simulink model "regulacja_pid"  (R2016b)
settings: Solver=VariableStepAuto  StartTime=0.0  StopTime=Tsym  RelTol=1e-3
undefined symbols (not defined in the file): D_12, D_21, decouplingEnabled, deltaFd, deltah, deltaT, deltaTc, deltaTd, deltaTh, disturbanceTime, enable_cross_tf, Fc_max, Fc_min, Fh_max, Fh_min, G1, h0, h_step_down_time, h_step_up_time, Kd, pid_ovation_h, pid_ovation_T, T0, T_step_down_time, T_step_up_time, Tp_pid
settings Model: Creator=Luke  LastModifiedBy=Luke

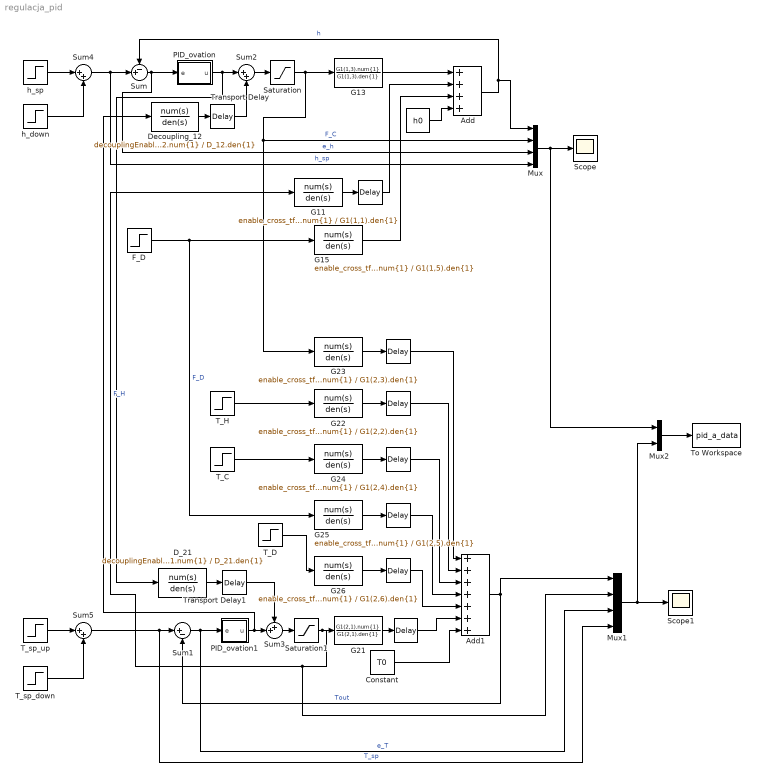
== system regulacja_pid ==
  " " : Constant  Value=h0
  "  " : TransportDelay  DelayTime=G1(2,1).ioDelay
  "   " : TransportDelay  DelayTime=G1(2,3).ioDelay
  "    " : TransportDelay  DelayTime=G1(2,2).ioDelay
  "     " : TransportDelay  DelayTime=G1(2,4).ioDelay
  "       " : TransportDelay  DelayTime=G1(2,5).ioDelay
  "        " : TransportDelay  DelayTime=G1(2,6).ioDelay
  "           " : TransportDelay  DelayTime=G1(1,1).IOdelay
  Add : Sum  Inputs=++++
  Add1 : Sum  Inputs=+++++++
  Constant : Constant  Value=T0
  D_21 : TransferFcn  Numerator=decouplingEnabled * D_21.num{1}  Denominator=D_21.den{1}
  Decoupling_12 : TransferFcn  Numerator=decouplingEnabled * D_12.num{1}  Denominator=D_12.den{1}
  F_D : Step  Time=1000  After=deltaFd  SampleTime=disturbanceTime
  G11 : TransferFcn  Numerator=enable_cross_tf * G1(1,1).num{1}  Denominator=G1(1,1).den{1}
  G13 : TransferFcn  Numerator=G1(1,3).num{1}  Denominator=G1(1,3).den{1}
  G15 : TransferFcn  Numerator=enable_cross_tf * G1(1,5).num{1}  Denominator=G1(1,5).den{1}
  G21 : TransferFcn  Numerator=G1(2,1).num{1}  Denominator=G1(2,1).den{1}
  G22 : TransferFcn  Numerator=enable_cross_tf * G1(2,2).num{1}  Denominator=G1(2,2).den{1}
  G23 : TransferFcn  Numerator=enable_cross_tf * G1(2,3).num{1}  Denominator=G1(2,3).den{1}
  G24 : TransferFcn  Numerator=enable_cross_tf * G1(2,4).num{1}  Denominator=G1(2,4).den{1}
  G25 : TransferFcn  Numerator=enable_cross_tf * G1(2,5).num{1}  Denominator=G1(2,5).den{1}
  G26 : TransferFcn  Numerator=enable_cross_tf * G1(2,6).num{1}  Denominator=G1(2,6).den{1}
  Mux : Mux
  Mux1 : Mux
  Mux2 : Mux  Inputs=2
  PID_ovation : Subsystem
  PID_ovation1 : Subsystem
  Saturation : Saturate  UpperLimit=Fc_max  LowerLimit=Fc_min
  Saturation1 : Saturate  UpperLimit=Fh_max  LowerLimit=Fh_min
  Scope : Scope
  Scope1 : Scope
  Sum : Sum  Inputs=-+|
  Sum1 : Sum  Inputs=|+-
  Sum2 : Sum  Inputs=|++
  Sum3 : Sum  Inputs=++|
  Sum4 : Sum  Inputs=|++
  Sum5 : Sum  Inputs=|++
  T_C : Step  After=deltaTc  SampleTime=0
  T_D : Step  After=deltaTd  SampleTime=0
  T_H : Step  After=deltaTh  SampleTime=0
  T_sp_down : Step  Time=T_step_down_time  After=-deltaT  SampleTime=0
  T_sp_up : Step  Time=T_step_up_time  Before=T0  After=T0+deltaT  SampleTime=0
  To Workspace : ToWorkspace  VariableName=pid_a_data  SaveFormat=Timeseries  SampleTime=-1
  Transport Delay : TransportDelay  DelayTime=D_12.IOdelay
  Transport Delay1 : TransportDelay  DelayTime=D_21.IOdelay
  h_down : Step  Time=h_step_down_time  After=-deltah  SampleTime=0
  h_sp : Step  Time=h_step_up_time  Before=h0  After=h0+deltah  SampleTime=0
  wires:
  " "/1 -> Add/4
  Add/1 -> Sum/1, Mux/1  "h"
  G13/1 -> Add/1
  PID_ovation/1(u) -> D_21/1, Sum2/1
  Sum/1 -> PID_ovation/1(e), Mux/3  "e_h"
  Sum4/1 -> Mux/4, Sum/2  "h_sp"
  Mux/1 -> Mux2/1, Scope/1
  G15/1 -> Add/3
  F_D/1 -> G25/1, G15/1  "F_D"
  Saturation1/1 -> G11/1, Mux1/2, G21/1  "F_H"
  Sum5/1 -> Mux1/4, Sum1/1  "T_sp"
  Sum1/1 -> PID_ovation1/1(e), Mux1/3  "e_T"
  Constant/1 -> Add1/7
  Add1/1 -> Mux1/1, Sum1/2  "Tout"
  "  "/1 -> Add1/6
  G21/1 -> "  "/1
  G26/1 -> "        "/1
  G24/1 -> "     "/1
  G25/1 -> "       "/1
  G22/1 -> "    "/1
  G23/1 -> "   "/1
  "        "/1 -> Add1/5
  "       "/1 -> Add1/4
  "     "/1 -> Add1/3
  "    "/1 -> Add1/2
  "   "/1 -> Add1/1
  T_H/1 -> G22/1
  T_C/1 -> G24/1
  T_D/1 -> G26/1
  Mux1/1 -> Mux2/2, Scope1/1
  Mux2/1 -> To Workspace/1
  Saturation/1 -> Mux/2, G23/1, G13/1  "F_C"
  Decoupling_12/1 -> Transport Delay/1
  Transport Delay/1 -> Sum2/2
  PID_ovation1/1(u) -> Decoupling_12/1, Sum3/2
  D_21/1 -> Transport Delay1/1
  Transport Delay1/1 -> Sum3/1
  h_sp/1 -> Sum4/1
  h_down/1 -> Sum4/2
  T_sp_down/1 -> Sum5/2
  T_sp_up/1 -> Sum5/1
  G11/1 -> "           "/1
  "           "/1 -> Add/2
  Sum2/1 -> Saturation/1
  Sum3/1 -> Saturation1/1

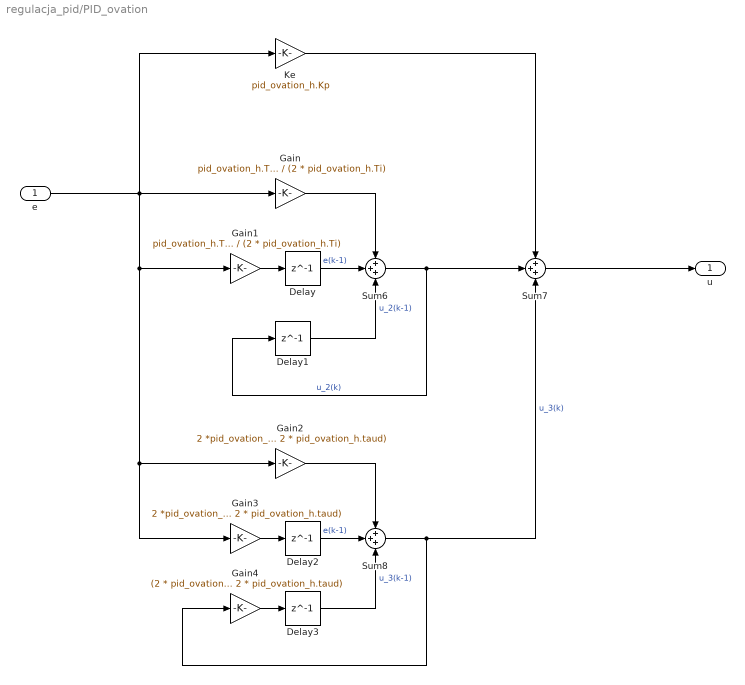
== system regulacja_pid/PID_ovation ==
  e : Inport
  Delay{,1..3} (4 alike) : Delay  DelayLength=1  SampleTime=Tp_pid
  Gain : Gain  Gain=pid_ovation_h.Tp / (2 * pid_ovation_h.Ti)
  Gain1 : Gain  Gain=pid_ovation_h.Tp / (2 * pid_ovation_h.Ti)
  Gain2 : Gain  Gain=2 *pid_ovation_h. Kd / (pid_ovation_h.Tp + 2 * pid_ovation_h.taud)
  Gain3 : Gain  Gain=2 *pid_ovation_h. Kd / (pid_ovation_h.Tp + 2 * pid_ovation_h.taud)
  Gain4 : Gain  Gain=(2 * pid_ovation_h.taud - pid_ovation_h.Tp) / (pid_ovation_h.Tp + 2 * pid_ovation_h.taud)
  Ke : Gain  Gain=pid_ovation_h.Kp
  Sum6 : Sum  Inputs=+++
  Sum7 : Sum  Inputs=+++
  Sum8 : Sum  Inputs=+++
  u : Outport
  wires:
  Delay3/1 -> Sum8/3  "u_3(k-1)"
  Gain3/1 -> Delay2/1
  e/1 -> Gain/1, Ke/1, Gain2/1, Gain3/1, Gain1/1
  Sum8/1 -> Sum7/3, Gain4/1  "u_3(k)"
  Delay2/1 -> Sum8/2  "e(k-1)"
  Gain2/1 -> Sum8/1
  Delay/1 -> Sum6/2  "e(k-1)"
  Delay1/1 -> Sum6/3  "u_2(k-1)"
  Gain/1 -> Sum6/1
  Sum6/1 -> Sum7/2, Delay1/1  "u_2(k)"
  Ke/1 -> Sum7/1
  Gain1/1 -> Delay/1
  Sum7/1 -> u/1
  Gain4/1 -> Delay3/1

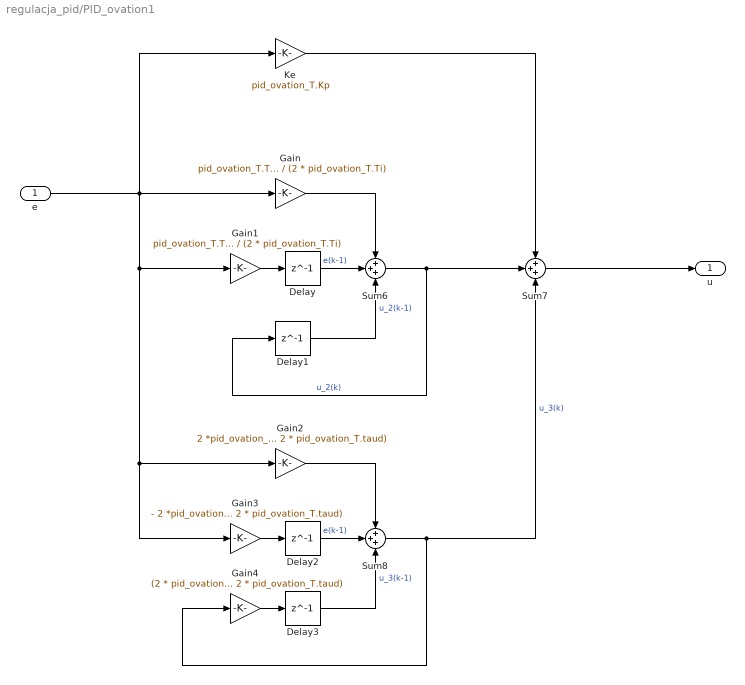
== system regulacja_pid/PID_ovation1 ==
  e : Inport
  Delay{,1..3} (4 alike) : Delay  DelayLength=1  SampleTime=Tp_pid
  Gain : Gain  Gain=pid_ovation_T.Tp / (2 * pid_ovation_T.Ti)
  Gain1 : Gain  Gain=pid_ovation_T.Tp / (2 * pid_ovation_T.Ti)
  Gain2 : Gain  Gain=2 *pid_ovation_T. Kd / (pid_ovation_T.Tp + 2 * pid_ovation_T.taud)
  Gain3 : Gain  Gain=- 2 *pid_ovation_T. Kd / (pid_ovation_T.Tp + 2 * pid_ovation_T.taud)
  Gain4 : Gain  Gain=(2 * pid_ovation_T.taud - pid_ovation_T.Tp) / (pid_ovation_T.Tp + 2 * pid_ovation_T.taud)
  Ke : Gain  Gain=pid_ovation_T.Kp
  Sum6 : Sum  Inputs=+++
  Sum7 : Sum  Inputs=+++
  Sum8 : Sum  Inputs=+++
  u : Outport
  wires:
  Delay3/1 -> Sum8/3  "u_3(k-1)"
  Gain3/1 -> Delay2/1
  e/1 -> Gain/1, Ke/1, Gain2/1, Gain3/1, Gain1/1
  Sum8/1 -> Sum7/3, Gain4/1  "u_3(k)"
  Delay2/1 -> Sum8/2  "e(k-1)"
  Gain2/1 -> Sum8/1
  Delay/1 -> Sum6/2  "e(k-1)"
  Delay1/1 -> Sum6/3  "u_2(k-1)"
  Gain/1 -> Sum6/1
  Sum6/1 -> Sum7/2, Delay1/1  "u_2(k)"
  Ke/1 -> Sum7/1
  Gain1/1 -> Delay/1
  Sum7/1 -> u/1
  Gain4/1 -> Delay3/1
